simulink model "mode_lame"  (R2020b)
settings: Solver=VariableStepAuto  StartTime=0.0  StopTime=10.0  RelTol=1e-3
settings Model: Creator=antoi  LastModifiedBy=antoi

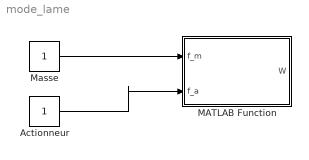
== system mode_lame ==
  Actionneur : Constant
  MATLAB Function : MATLAB Function  TreatAsAtomicUnit=on
  Masse : Constant
  wires:
  Masse/1 -> MATLAB Function/1(f_m)
  Actionneur/1 -> MATLAB Function/2(f_a)

== matlab function mode_lame/MATLAB Function ==
  data: f_m input; W output; f_a input
function W = fcn(f_m, f_a)
    global w_old w coeff1 coeff2 coeff3 coeff4 g; 
    
    % Vecteur position
    w_new = zeros(1,nx);
    
    % Amortissement
    B = 6; % Ajuster l'amortissement
    
    
    % Calcul des coeff
    coeff3 = B/(dt);
    coeff4 = ((mu/dt^2) + (B/dt))^(-1);
    
    % Force
    f_m = -g*m;
    
    f = zeros(1, nx);
    f(9:11) = (f_m + f_a)/3;
    
    
    i = 3:nx-2;
    %Équation différentielle résolue par Sam
    w_new(i) = (-coeff1*(w(i+2)-4*w(i+1)+6*w(i)-4*w(i-1)+w(i-2)) - coeff2*(-2*w(i)+w_old(i)) + coeff3*w(i) + f(i)/dx_n)*coeff4;
    
    %% Conditions limites 
 
     w_new(1:2) =0;                 % Clampé à zero, position et dérivée nulle (le bout de la lame est fixe)
   
     w_new(end-1) = 2*w_new(end-2)-w_new(end-3);    % Libre au bout dérivées 2e et 3e nulles
     w_new(end) = 2*w_new(end-1)-w_new(end-2);
     
    %% Préparation du prochain tour
    
    w_old = w;
    w = w_new;
    
    W = w(end);
